simulink model "VSC"  (R2019b)
settings: Solver=ode23tb  StartTime=0.0  StopTime=0.2  MaxStep=5e-6  RelTol=1e-3  AbsTol=.01  EnableMultiTasking=on
libraries: powerlib x12, powerlib_meascontrol x1, simulink x1
settings Model: Creator=Lenovo  LastModifiedBy=96547
settings SolverCC: AutoScaleAbsTol=off
settings DataIOCC: LimitDataPoints=on  SaveFormat=Array  SignalLoggingSaveFormat=ModelDataLogs  ReturnWorkspaceOutputs=off
settings OptimizationCC: InitFltsAndDblsToZero=on  LifeSpan=inf
settings DebuggingCC: SaveWithParameterizedLinksMsg=none  UnderspecifiedInitializationDetection=Classic  MergeDetectMultiDrivingBlocksExec=none  SignalResolutionControl=TryResolveAllWithWarning  SolverPrmCheckMsg=warning  MultiTaskDSMMsg=warning  MultiTaskCondExecSysMsg=none  FcnCallInpInsideContextMsg=warning  SFUnexpectedBacktrackingDiag=warning  SFNoUnconditionalDefaultTransitionDiag=warning  SFExecutionAtInitializationDiag=none  ArithmeticOperatorsInVariantConditions=warning
settings HardwareCC: ProdBitPerPointer=32  ProdBitPerSizeT=32  ProdBitPerPtrDiffT=32  ProdLargestAtomicFloat=None  ProdIntDivRoundTo=Undefined  ProdEndianess=Unspecified  ProdWordSize=32  ProdHWDeviceType=32-bit Generic
settings ModelReferenceCC: PropagateSignalLabelsOutOfModel=off
settings CodeAppCC: StateflowObjectComments=on
settings GRTTargetCC: TargetFcnLib=ansi_tfl_tmw.mat  TargetLangStandard=C89/C90 (ANSI)  CombineOutputUpdateFcns=off  GRTInterface=on
settings ConfigComp: CovMetricSettings=dw  CovHtmlReporting=on  CovSaveCumulativeToWorkspaceVar=on  CovSaveSingleToWorkspaceVar=on

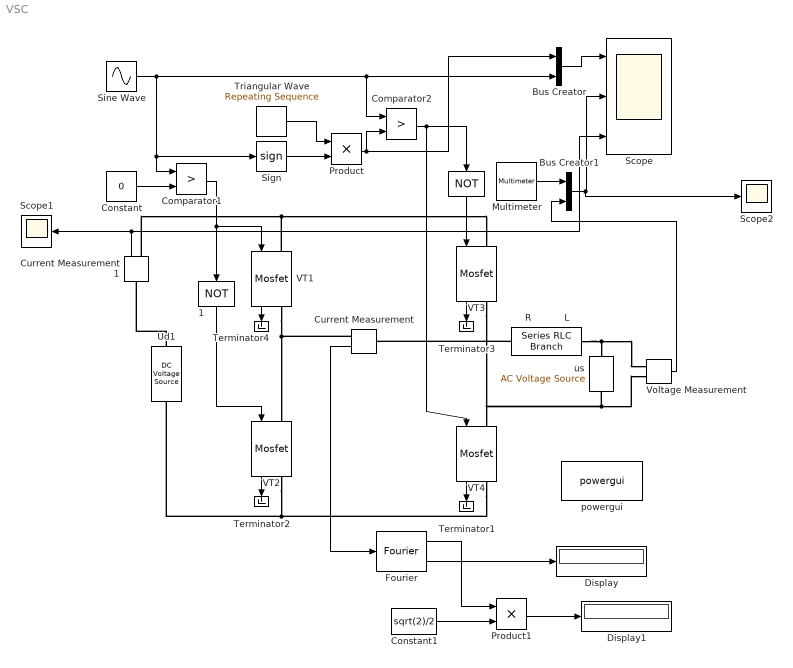
== system VSC ==
  " " : Logic  Operator=NOT  AllPortsSameDT=off  OutDataTypeStr=boolean
  " 1" : Logic  Operator=NOT  AllPortsSameDT=off  OutDataTypeStr=boolean
  Bus Creator : BusCreator  DialogController=Simulink.DDGSource_Bus  Inputs=2
  Bus Creator1 : BusCreator  DialogController=Simulink.DDGSource_Bus  Inputs=2
  Comparator1 : RelationalOperator  Operator=>  OutDataTypeStr=boolean  ZeroCross=off  RndMeth=Nearest
  Comparator2 : RelationalOperator  Operator=>  OutDataTypeStr=boolean  ZeroCross=off  RndMeth=Nearest
  Constant : Constant  Value=0
  Constant1 : Constant  Value=sqrt(2)/2
  Current Measurement : powerlib/Measurements/Current Measurement  PhasorSimulation=off  OutputType=Complex  PSBequivalent=0
      settings: SourceProductName=Simscape Electrical
  Current Measurement1 : powerlib/Measurements/Current Measurement  PhasorSimulation=off  OutputType=Complex  PSBequivalent=0
      settings: SourceProductName=Simscape Electrical
  Display : Display
  Display1 : Display
  Fourier : powerlib_meascontrol/Measurements/Fourier  Freq=60  n=1  InInit=[0, 0]  Ts=0
      settings: SourceProductName=Simscape Electrical
  Multimeter : powerlib/Measurements/Multimeter  PhasorSimulation=off  OutputType=Complex  sel=2  L=2  Gain=1  yselected="{'Ib: R           L'};"  PSBOutputType=1  PSBequivalent=0  AxesSetting=[0,0.1,-100,100]  Display=0  SavedBlockNames=-11
      settings: SourceProductName=Simscape Electrical
  Product : Product  RndMeth=Zero
  Product1 : Product  RndMeth=Zero
  R           L : powerlib/Elements/Series RLC Branch  LConnTagsString=__new0  RConnTagsString=__new0  BranchType=RL  Resistance=0.1  Inductance=0.006  SetiL0=off  InitialCurrent=0  Capacitance=inf  Setx0=off  InitialVoltage=0  Measurements=Branch voltage and current
      settings: SourceProductName=Simscape Electrical
  Scope : Scope  NumInputPorts=3
  Scope1 : Scope
  Scope2 : Scope
  Sign : Signum
  Sine Wave : Sin  Amplitude=0.590025  Frequency=2*pi*50  Phase=0.0814685  SampleTime=0
  Terminator{1..4} (4 alike) : Terminator
  Triangular Wave : simulink/Sources/Repeating Sequence  rep_seq_t=[0 2.5e-5 5e-5]  rep_seq_y=[1 0 1]
  Ud1 : powerlib/Electrical Sources/DC Voltage Source  Amplitude=640  Measurements=None
      settings: SourceProductName=Simscape Electrical
  VT1 : powerlib/Power Electronics/Mosfet  Ron=0.01  Lon=1e-7  Rd=.01  Vfd=0  IC=0  Rs=5  Cs=1e-6  Measurements=on
      settings: SourceProductName=Simscape Electrical
  VT2 : powerlib/Power Electronics/Mosfet  Ron=0  Lon=1e-7  Rd=0  Vfd=0  IC=0  Rs=5  Cs=1e-6  Measurements=on
      settings: SourceProductName=Simscape Electrical
  VT3 : powerlib/Power Electronics/Mosfet  Ron=0  Lon=1e-7  Rd=0  Vfd=0  IC=0  Rs=5  Cs=1e-6  Measurements=on
      settings: SourceProductName=Simscape Electrical
  VT4 : powerlib/Power Electronics/Mosfet  Ron=0  Lon=1e-7  Rd=0  Vfd=0  IC=0  Rs=5  Cs=1e-6  Measurements=on
      settings: SourceProductName=Simscape Electrical
  Voltage Measurement : powerlib/Measurements/Voltage Measurement  PhasorSimulation=off  OutputType=Complex  PSBequivalent=0
      settings: SourceProductName=Simscape Electrical
  powergui : powerlib/powergui  Priority=1  SimulationMode=Continuous  SampleTime=50e-6  frequency=60  Iterations=50  frequencyindice=0  Pbase=100e6  ErrMax=1e-4  UnitsV=kV  UnitsW=MW  buscounter=0  FunctionMessages=off  echomessages=off  EnableUseOfTLC=off  CurrentSourceSwitches=off  DisableSnubberDevices=off  DisableRonSwitches=off  DisableVfSwitches=off  DisplayEquations=off  AutomaticDiscreteSolvers=off  SolverType=Tustin/Backward Euler (TBE)  Interpol=off  ExternalGateDelay=off  methode=off  Ts=100  x0status=blocks  SPID=on  SwTol=0  HookPort=off  NonlinearTolerance=1e-4  nMaxIteration=100  ContinueOnMaxIteration=off  RestoreLinks=warning  ResistiveCurrentMeasurement=off  Frange=[0:2:500]  Ylog=off  Xlog=on  ShowGrid=off  save=off  variable=ZData  structure=0  ZoomFFT=off  StartTime=0.0  cycles=1  DisplayStyle=1  fundamental=60  FreqAxis=off  MaxFrequency=1000  frequencyindicesteady=1  RmsSteady=1  display=off
      settings: SourceProductName=Simscape Electrical
  us : powerlib/Electrical Sources/AC Voltage Source  Amplitude=220*sqrt(2)  Phase=0  Frequency=50  SampleTime=0  Measurements=None  BusType=swing  Pref=10e3  Qref=0  Qmin=-inf  Qmax=+inf
      settings: SourceProductName=Simscape Electrical
  wires:
  Comparator2/1 -> " "/1, VT4/1
  VT4/1 -> Terminator1/1
  VT2/1 -> Terminator2/1
  VT3/1 -> Terminator3/1
  Sine Wave/1 -> Sign/1, Comparator1/1, Comparator2/1, Bus Creator/2
  Bus Creator/1 -> Scope/1
  " "/1 -> VT3/1
  Sign/1 -> Product/2
  " 1"/1 -> VT2/1
  Triangular Wave/1 -> Product/1
  Product/1 -> Bus Creator/1, Comparator2/2
  Comparator1/1 -> VT1/1, " 1"/1
  Constant/1 -> Comparator1/2
  Multimeter/1 -> Bus Creator1/1
  Voltage Measurement/1 -> Bus Creator1/2
  Bus Creator1/1 -> Scope2/1, Scope/2
  VT1/1 -> Terminator4/1
  Current Measurement/1 -> Fourier/1
  Fourier/2 -> Display/1
  Fourier/1 -> Product1/1
  Constant1/1 -> Product1/2
  Product1/1 -> Display1/1
  Current Measurement1/1 -> Scope1/1, Scope/3
  connections:
  VT3/RConn1 -- VT4/LConn1 -- us/LConn1 -- Voltage Measurement/LConn2
  VT1/RConn1 -- Current Measurement/RConn1 -- VT2/LConn1
  VT4/RConn1 -- Ud1/LConn1 -- VT2/RConn1
  VT1/LConn1 -- Current Measurement1/RConn1 -- VT3/LConn1
  R           L/RConn1 -- us/RConn1 -- Voltage Measurement/LConn1
  R           L/LConn1 -- Current Measurement/LConn1
  Ud1/RConn1 -- Current Measurement1/LConn1
